simulink model "quad_eom"  (R2021a)
settings: Solver=VariableStepAuto  StartTime=0.0  StopTime=10  RelTol=1e-3
undefined symbols (not defined in the file or in its folder): eul_0, eul_init, g, I, m, pm_0, Vb_init, Vm_0, wb_init, Xe_init, xme_0
libraries: simulink_extras x3
settings Model: Creator=Petronas-Tareq  LastModifiedBy=Petronas-Tareq

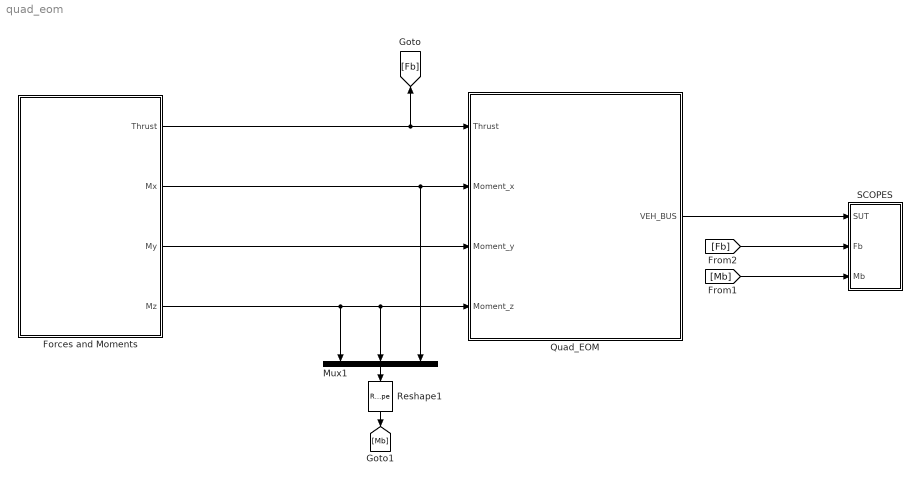
== system quad_eom ==
  Forces and Moments : Subsystem  Variant=on  VariantControlMode=label  LabelModeActiveChoice=free_fall
  Mux1 : Mux  Inputs=3
  Quad_EOM : Subsystem
      mask Display: image('$imagefile'); % Use "Edit Image" on toolstrip to change.
  Reshape1 : Reshape  OutputDimensionality=Column vector (2-D)
  SCOPES : Subsystem
  wires:
  Mux1/1 -> Reshape1/1
  Reshape1/1 -> [Mb]
  [Mb] -> SCOPES/3(Mb)
  [Fb] -> SCOPES/2(Fb)
  Quad_EOM/1(VEH_BUS) -> SCOPES/1(SUT)
  Forces and Moments/1(Thrust) -> Quad_EOM/1(Thrust), [Fb]
  Forces and Moments/2(Mx) -> Quad_EOM/2(Moment_x), Mux1/3
  Forces and Moments/3(My) -> Quad_EOM/3(Moment_y)
  Forces and Moments/4(Mz) -> Mux1/1, Quad_EOM/4(Moment_z), Mux1/2

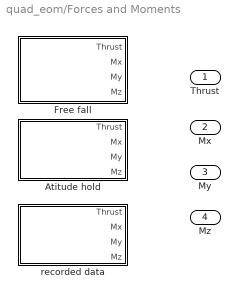
== system quad_eom/Forces and Moments ==
  Atitude hold : Subsystem  VariantControl=Alt_hold
  Free fall : Subsystem  VariantControl=free_fall
  recorded data : Subsystem  VariantControl=recorded
  Thrust : Outport
  Mx : Outport  Port=2
  My : Outport  Port=3
  Mz : Outport  Port=4

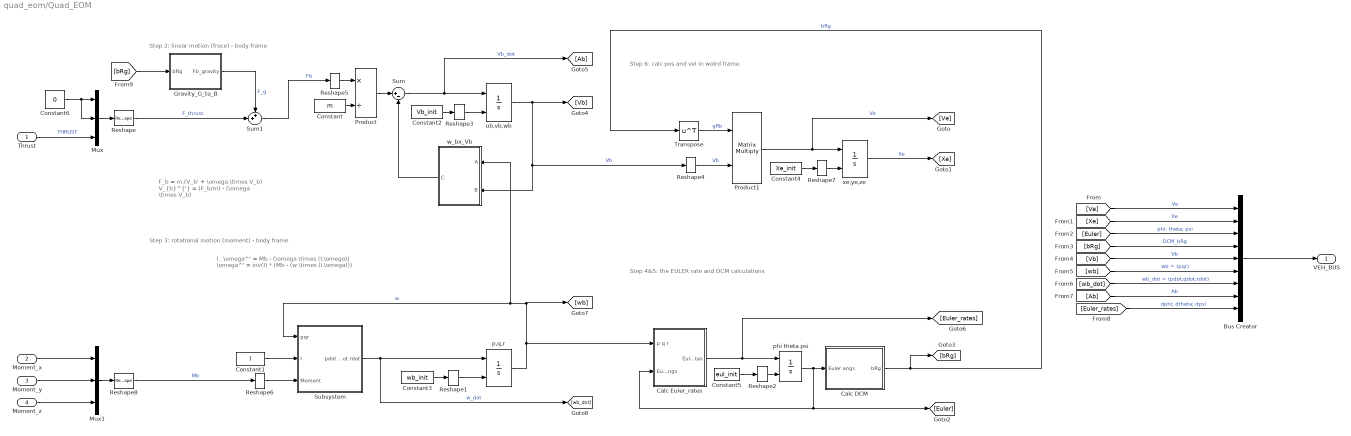
== system quad_eom/Quad_EOM ==
  note: Step 3: rotational motion (moment) - body frame
  note: F_b = m.(V_b' + \omega \times V_b)
      |
      | V_{b}^{'} = (F_b/m) - (\omega \times V_b)
  note: Step 2: linear motion (froce) - body frame
  note: Step 6: calc pos and vel in wolrd frame
  note: I . \omega^' = Mb - (\omega \times (I.\omega))
      |
      | \omega^' = inv(I) * (Mb - (w \times (I.\omega)))
  note: Step 4&5: the EULER rate and DCM calculations
  Thrust : Inport
  Moment_x : Inport  Port=2
  Moment_y : Inport  Port=3
  Moment_z : Inport  Port=4
  Bus Creator : BusCreator  Inputs=9
  Calc DCM : Subsystem
  Calc Euler_rates : Subsystem
  Constant : Constant  Value=m  OutDataTypeStr=Inherit: Inherit via back propagation
  Constant1 : Constant  Value=I  OutDataTypeStr=Inherit: Inherit via back propagation
  Constant2 : Constant  Value=Vb_init  OutDataTypeStr=Inherit: Inherit via back propagation
  Constant3 : Constant  Value=wb_init  OutDataTypeStr=Inherit: Inherit via back propagation
  Constant4 : Constant  Value=Xe_init  OutDataTypeStr=Inherit: Inherit via back propagation
  Constant5 : Constant  Value=eul_init  OutDataTypeStr=Inherit: Inherit via back propagation
  Constant6 : Constant  Value=0
  Gravity_G_to_B : Subsystem
  Mux : Mux  Inputs=3
  Mux1 : Mux  Inputs=3
  Product : Product  Inputs=*/  SaturateOnIntegerOverflow=on  OutDataTypeStr=Inherit: Same as first input
  Product1 : Product  Multiplication=Matrix(*)  InputSameDT=on  SaturateOnIntegerOverflow=on  OutDataTypeStr=Inherit: Same as first input
  Reshape{,1..8} (9 alike) : Reshape  OutputDimensionality=Column vector (2-D)
  Subsystem : Subsystem
  Sum : Sum  Inputs=|+-  SaturateOnIntegerOverflow=on
  Sum1 : Sum  Inputs=++|
  Transpose : Math  Operator=transpose  SignedPower=on  SaturateOnIntegerOverflow=on
  "p,q,r " : Integrator  InitialConditionSource=external  InitialCondition=pm_0
  phi theta psi : Integrator  InitialConditionSource=external  InitialCondition=eul_0
  ub,vb,wb : Integrator  InitialConditionSource=external  InitialCondition=Vm_0
  w_bx_Vb : Subsystem
      mask Display:
      | text(.5,.5,'Cross\nProduct\n\nC = AxB', ...
      | 	'HorizontalAlignment','Center',...
      | 	'VerticalAlignment','middle')
  xe,ye,ze : Integrator  InitialConditionSource=external  InitialCondition=xme_0
  VEH_BUS : Outport  VectorParamsAs1DForOutWhenUnconnected=off
  wires:
  [Euler] -> Bus Creator/3  "phi; theta; psi"
  [Xe] -> Bus Creator/2  "Xe"
  [Ve] -> Bus Creator/1  "Ve"
  [bRg] -> Bus Creator/4  "DCM_bRg"
  [Ab] -> Bus Creator/8  "Ab"
  [wb_dot] -> Bus Creator/7  "wb_dot = (pdot;qdot;rdot)"
  Bus Creator/1 -> VEH_BUS/1
  [Vb] -> Bus Creator/5  "Vb"
  [wb] -> Bus Creator/6  "wb = (pqr)"
  [Euler_rates] -> Bus Creator/9  "dphi; dtheta; dpsi"
  Reshape8/1 -> Reshape6/1  "Mb"
  Reshape6/1 -> Subsystem/3(Moment)
  Constant5/1 -> Reshape2/1
  Reshape1/1 -> "p,q,r "/2
  phi theta psi/1 -> Calc DCM/1(Euler angs), Calc Euler_rates/2(Euler_angs), [Euler]
  Transpose/1 -> Product1/1  "gRb"
  Constant2/1 -> Reshape3/1
  ub,vb,wb/1 -> w_bx_Vb/2(B), Reshape4/1, [Vb]  "Vb"
  Subsystem/1(pdot qdot rdot) -> [wb_dot], "p,q,r "/1  "w_dot"
  Constant/1 -> Product/2
  Constant1/1 -> Subsystem/2(I)
  Reshape4/1 -> Product1/2  "Vb"
  w_bx_Vb/1(C) -> Sum/2
  Calc DCM/1(bRg) -> [bRg], Transpose/1  "bRg"
  Calc Euler_rates/1(Euler_rates) -> [Euler_rates], phi theta psi/1
  Reshape2/1 -> phi theta psi/2
  Sum/1 -> [Ab], ub,vb,wb/1  "Vb_dot"
  Constant4/1 -> Reshape7/1
  Reshape3/1 -> ub,vb,wb/2
  "p,q,r "/1 -> [wb], Subsystem/1(pqr), w_bx_Vb/1(A), Calc Euler_rates/1("p q r ")  "w"
  Reshape7/1 -> xe,ye,ze/2
  Product1/1 -> [Ve], xe,ye,ze/1  "Ve"
  Reshape5/1 -> Product/1
  xe,ye,ze/1 -> [Xe]  "Xe"
  Sum1/1 -> Reshape5/1  "Fb"
  Constant3/1 -> Reshape1/1
  Product/1 -> Sum/1
  Constant6/1 -> Mux/2, Mux/1
  Gravity_G_to_B/1(Fb_gravity) -> Sum1/1  "F_g"
  Mux/1 -> Reshape/1
  Reshape/1 -> Sum1/2  "F_thrust"
  Thrust/1 -> Mux/3  "THRUST"
  [bRg] -> Gravity_G_to_B/1(bRg)
  Moment_y/1 -> Mux1/2
  Moment_z/1 -> Mux1/3
  Mux1/1 -> Reshape8/1
  Moment_x/1 -> Mux1/1

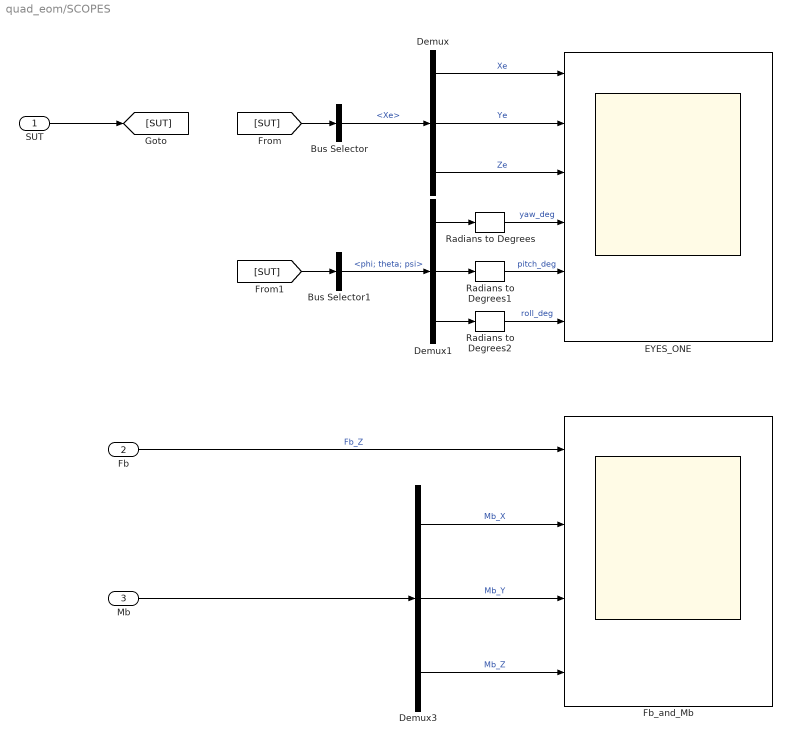
== system quad_eom/SCOPES ==
  SUT : Inport
  Fb : Inport  Port=2
  Mb : Inport  Port=3
  Bus Selector : BusSelector  OutputSignals=Xe
  Bus Selector1 : BusSelector  OutputSignals=phi; theta; psi
  Demux : Demux  Outputs=3
  Demux1 : Demux  Outputs=3
  Demux3 : Demux  Outputs=3
  EYES_ONE : Scope  NumInputPorts=6
  Fb_and_Mb : Scope  NumInputPorts=4
  Radians to Degrees : simulink_extras/Transformations/Radians to Degrees
  Radians to Degrees1 : simulink_extras/Transformations/Radians to Degrees
  Radians to Degrees2 : simulink_extras/Transformations/Radians to Degrees
  wires:
  SUT/1 -> [SUT]
  [SUT] -> Bus Selector/1
  Demux/2 -> EYES_ONE/2  "Ye"
  Demux/3 -> EYES_ONE/3  "Ze"
  Demux/1 -> EYES_ONE/1  "Xe"
  Bus Selector/1 -> Demux/1  "<Xe>"
  Bus Selector1/1 -> Demux1/1  "<phi; theta; psi>"
  [SUT] -> Bus Selector1/1
  Demux1/1 -> Radians to Degrees/1
  Radians to Degrees/1 -> EYES_ONE/4  "yaw_deg"
  Radians to Degrees1/1 -> EYES_ONE/5  "pitch_deg"
  Radians to Degrees2/1 -> EYES_ONE/6  "roll_deg"
  Demux1/3 -> Radians to Degrees2/1
  Demux1/2 -> Radians to Degrees1/1
  Fb/1 -> Fb_and_Mb/1  "Fb_Z"
  Mb/1 -> Demux3/1
  Demux3/1 -> Fb_and_Mb/2  "Mb_X"
  Demux3/2 -> Fb_and_Mb/3  "Mb_Y"
  Demux3/3 -> Fb_and_Mb/4  "Mb_Z"

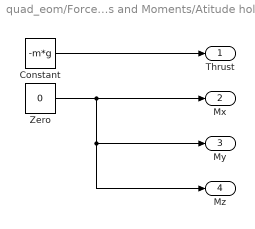
== system quad_eom/Forces and Moments/Atitude hold ==
  Constant : Constant  Value=-m*g
  Zero : Constant  Value=0  OutDataTypeStr=Inherit: Inherit via back propagation
  Thrust : Outport
  Mx : Outport  Port=2
  My : Outport  Port=3
  Mz : Outport  Port=4
  wires:
  Constant/1 -> Thrust/1
  Zero/1 -> Mz/1, My/1, Mx/1

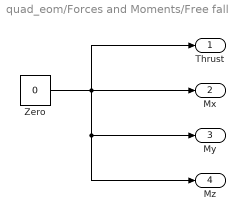
== system quad_eom/Forces and Moments/Free fall ==
  Zero : Constant  Value=0  OutDataTypeStr=Inherit: Inherit via back propagation
  Thrust : Outport
  Mx : Outport  Port=2
  My : Outport  Port=3
  Mz : Outport  Port=4
  wires:
  Zero/1 -> Thrust/1, Mx/1, My/1, Mz/1

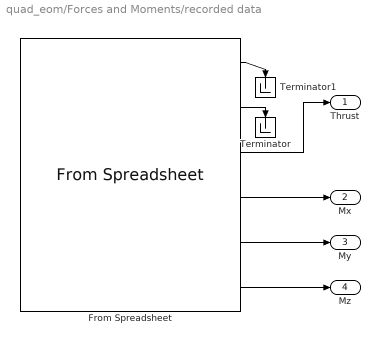
== system quad_eom/Forces and Moments/recorded data ==
  From Spreadsheet : FromSpreadsheet  FileName=FbMb_data.xlsx  SheetName=D_short_XYZ  ExtrapolationAfterLastDataPoint=Hold last value
  Terminator : Terminator
  Terminator1 : Terminator
  Thrust : Outport
  Mx : Outport  Port=2
  My : Outport  Port=3
  Mz : Outport  Port=4
  wires:
  From Spreadsheet/1 -> Terminator1/1
  From Spreadsheet/3 -> Thrust/1
  From Spreadsheet/5 -> My/1
  From Spreadsheet/2 -> Terminator/1
  From Spreadsheet/4 -> Mx/1
  From Spreadsheet/6 -> Mz/1

== system quad_eom/Quad_EOM/Calc DCM ==
  Euler angs : Inport
  Calculate DCM bRw : MATLAB Function  TreatAsAtomicUnit=on
  Demux3 : Demux  Outputs=3
  bRg : Outport
  wires:
  Calculate DCM bRw/1(bRw) -> bRg/1
  Demux3/2 -> Calculate DCM bRw/2(theta_t)  "thetsa"
  Demux3/3 -> Calculate DCM bRw/3(psi_t)  "psi"
  Demux3/1 -> Calculate DCM bRw/1(phi_t)  "phi"
  Euler angs/1 -> Demux3/1

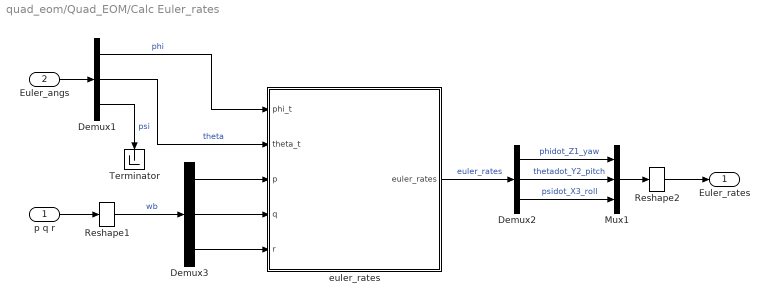
== system quad_eom/Quad_EOM/Calc Euler_rates ==
  "p q r " : Inport
  Euler_angs : Inport  Port=2
  Demux1 : Demux  Outputs=3
  Demux2 : Demux  Outputs=3
  Demux3 : Demux  Outputs=3
  Mux1 : Mux  Inputs=3
  Reshape1 : Reshape  OutputDimensionality=Column vector (2-D)
  Reshape2 : Reshape  OutputDimensionality=Column vector (2-D)
  Terminator : Terminator
  euler_rates : MATLAB Function  TreatAsAtomicUnit=on
  Euler_rates : Outport
  wires:
  Demux2/2 -> Mux1/2  "thetadot_Y2_pitch"
  Demux1/1 -> euler_rates/1(phi_t)  "phi"
  Demux3/2 -> euler_rates/4(q)
  Demux2/1 -> Mux1/1  "phidot_Z1_yaw"
  "p q r "/1 -> Reshape1/1
  Euler_angs/1 -> Demux1/1
  Demux3/1 -> euler_rates/3(p)
  Reshape2/1 -> Euler_rates/1
  Reshape1/1 -> Demux3/1  "wb"
  Demux3/3 -> euler_rates/5(r)
  Demux1/3 -> Terminator/1  "psi"
  euler_rates/1(euler_rates) -> Demux2/1  "euler_rates"
  Demux1/2 -> euler_rates/2(theta_t)  "theta"
  Mux1/1 -> Reshape2/1
  Demux2/3 -> Mux1/3  "psidot_X3_roll"

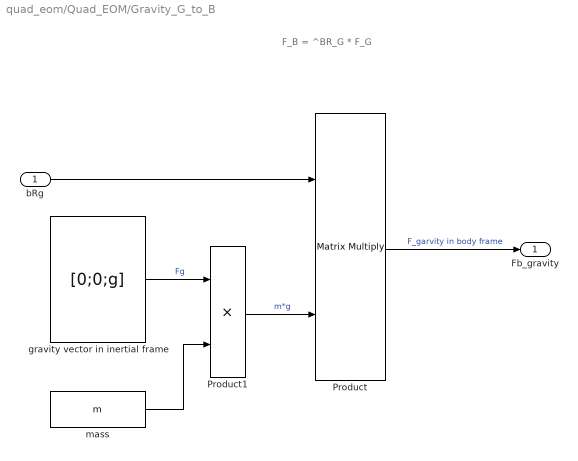
== system quad_eom/Quad_EOM/Gravity_G_to_B ==
  note: F_B = ^BR_G * F_G
  bRg : Inport
  Product : Product  Multiplication=Matrix(*)
  Product1 : Product
  gravity vector in inertial frame : Constant  Value=[0;0;g]  VectorParams1D=off
  mass : Constant  Value=m
  Fb_gravity : Outport  VectorParamsAs1DForOutWhenUnconnected=off
  wires:
  bRg/1 -> Product/1
  Product/1 -> Fb_gravity/1  "F_garvity in body frame"
  Product1/1 -> Product/2  "m*g"
  gravity vector in inertial frame/1 -> Product1/1  "Fg"
  mass/1 -> Product1/2

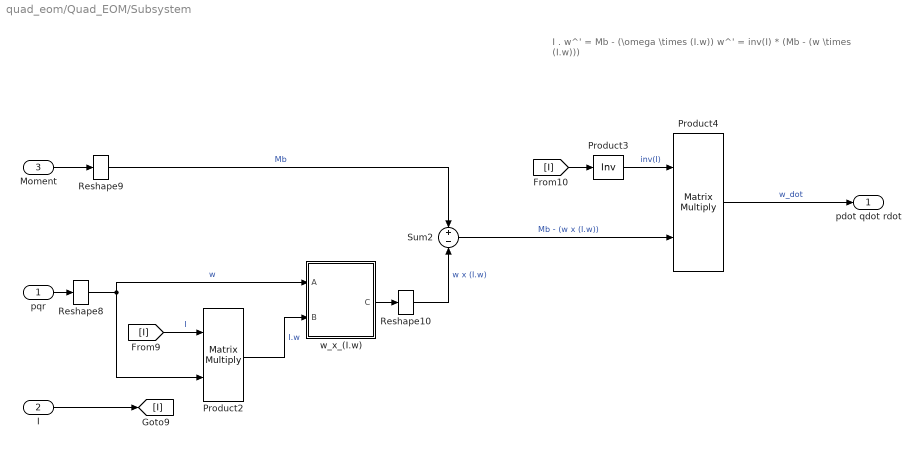
== system quad_eom/Quad_EOM/Subsystem ==
  note: I . w^' = Mb - (\omega \times (I.w))
      |
      | w^' = inv(I) * (Mb - (w \times (I.w)))
  pqr : Inport
  I : Inport  Port=2
  Moment : Inport  Port=3
  Product2 : Product  Multiplication=Matrix(*)  InputSameDT=on  SaturateOnIntegerOverflow=on  OutDataTypeStr=Inherit: Same as first input
  Product3 : Product  Inputs=/  Multiplication=Matrix(*)  SaturateOnIntegerOverflow=on  OutDataTypeStr=Inherit: Same as first input
  Product4 : Product  Multiplication=Matrix(*)  SaturateOnIntegerOverflow=on  OutDataTypeStr=Inherit: Same as first input
  Reshape10 : Reshape  OutputDimensionality=Column vector (2-D)
  Reshape8 : Reshape  OutputDimensionality=Column vector (2-D)
  Reshape9 : Reshape  OutputDimensionality=Column vector (2-D)
  Sum2 : Sum  Inputs=+|-  SaturateOnIntegerOverflow=on
  w_x_(I.w) : Subsystem
      mask Display:
      | text(.5,.5,'Cross\nProduct\n\nC = AxB', ...
      | 	'HorizontalAlignment','Center',...
      | 	'VerticalAlignment','middle')
  pdot qdot rdot : Outport
  wires:
  Product2/1 -> w_x_(I.w)/2(B)  "I.w"
  Product3/1 -> Product4/1  "inv(I)"
  Reshape8/1 -> w_x_(I.w)/1(A), Product2/2  "w"
  [I] -> Product3/1
  pqr/1 -> Reshape8/1
  Reshape9/1 -> Sum2/1  "Mb"
  Sum2/1 -> Product4/2  "Mb - (w x (I.w))"
  Reshape10/1 -> Sum2/2  "w x (I.w)"
  w_x_(I.w)/1(C) -> Reshape10/1
  [I] -> Product2/1  "I"
  Product4/1 -> pdot qdot rdot/1  "w_dot"
  Moment/1 -> Reshape9/1
  I/1 -> [I]

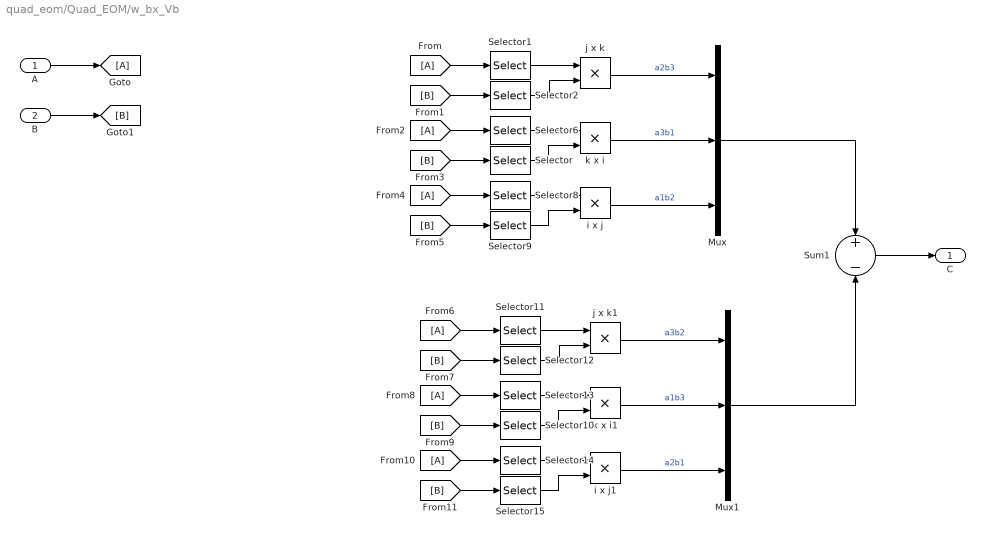
== system quad_eom/Quad_EOM/w_bx_Vb ==
  A : Inport
  B : Inport  Port=2
  Mux : Mux  Inputs=3
  Mux1 : Mux  Inputs=3
  Selector{,8,13,15} (4 alike) : Selector  InputPortWidth=3  IndexOptions=Index vector (dialog)  Indices=1  OutputSizes=1
  Selector{1,9,12,14} (4 alike) : Selector  InputPortWidth=3  IndexOptions=Index vector (dialog)  Indices=2  OutputSizes=1
  Selector{2,6,10..11} (4 alike) : Selector  InputPortWidth=3  IndexOptions=Index vector (dialog)  Indices=3  OutputSizes=1
  Sum1 : Sum  Inputs=+|-  InputSameDT=on  SaturateOnIntegerOverflow=on  OutDataTypeStr=Inherit: Same as first input
  i x j : Product  InputSameDT=on  SaturateOnIntegerOverflow=on  OutDataTypeStr=Inherit: Same as first input
  i x j1 : Product  InputSameDT=on  SaturateOnIntegerOverflow=on  OutDataTypeStr=Inherit: Same as first input
  j x k : Product  InputSameDT=on  SaturateOnIntegerOverflow=on  OutDataTypeStr=Inherit: Same as first input
  j x k1 : Product  InputSameDT=on  SaturateOnIntegerOverflow=on  OutDataTypeStr=Inherit: Same as first input
  k x i : Product  InputSameDT=on  SaturateOnIntegerOverflow=on  OutDataTypeStr=Inherit: Same as first input
  k x i1 : Product  InputSameDT=on  SaturateOnIntegerOverflow=on  OutDataTypeStr=Inherit: Same as first input
  C : Outport
  wires:
  i x j/1 -> Mux/3  "a1b2"
  k x i/1 -> Mux/2  "a3b1"
  j x k/1 -> Mux/1  "a2b3"
  Mux/1 -> Sum1/1
  Sum1/1 -> C/1
  Selector1/1 -> j x k/1
  Selector2/1 -> j x k/2
  B/1 -> [B]
  A/1 -> [A]
  [B] -> Selector2/1
  [A] -> Selector1/1
  [A] -> Selector6/1
  [B] -> Selector/1
  Selector6/1 -> k x i/1
  Selector/1 -> k x i/2
  [A] -> Selector8/1
  [B] -> Selector9/1
  Selector8/1 -> i x j/1
  Selector9/1 -> i x j/2
  i x j1/1 -> Mux1/3  "a2b1"
  k x i1/1 -> Mux1/2  "a1b3"
  j x k1/1 -> Mux1/1  "a3b2"
  Mux1/1 -> Sum1/2
  Selector11/1 -> j x k1/1
  Selector12/1 -> j x k1/2
  [B] -> Selector12/1
  [A] -> Selector11/1
  [A] -> Selector13/1
  [B] -> Selector10/1
  Selector13/1 -> k x i1/1
  Selector10/1 -> k x i1/2
  [A] -> Selector14/1
  [B] -> Selector15/1
  Selector14/1 -> i x j1/1
  Selector15/1 -> i x j1/2

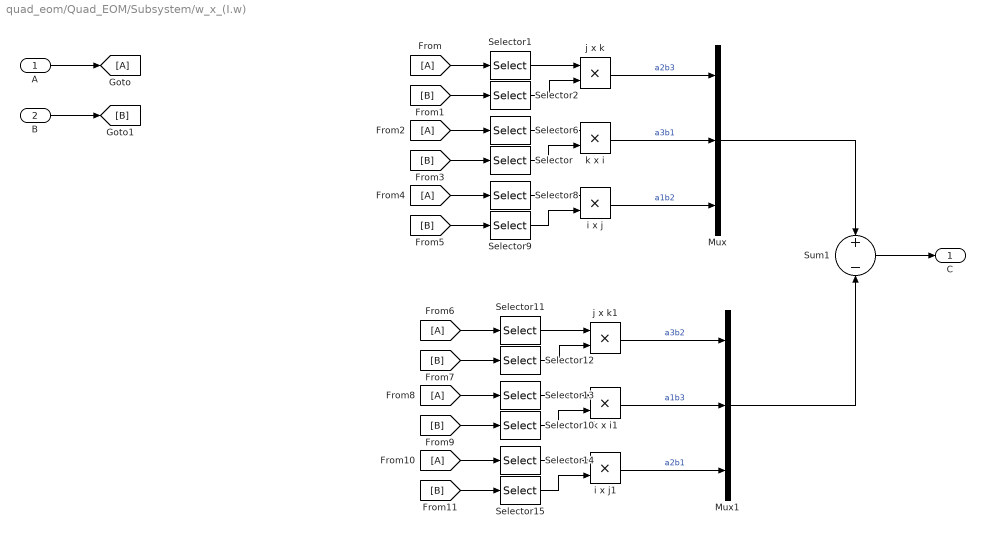
== system quad_eom/Quad_EOM/Subsystem/w_x_(I.w) ==
  A : Inport
  B : Inport  Port=2
  Mux : Mux  Inputs=3
  Mux1 : Mux  Inputs=3
  Selector{,8,13,15} (4 alike) : Selector  InputPortWidth=3  IndexOptions=Index vector (dialog)  Indices=1  OutputSizes=1
  Selector{1,9,12,14} (4 alike) : Selector  InputPortWidth=3  IndexOptions=Index vector (dialog)  Indices=2  OutputSizes=1
  Selector{2,6,10..11} (4 alike) : Selector  InputPortWidth=3  IndexOptions=Index vector (dialog)  Indices=3  OutputSizes=1
  Sum1 : Sum  Inputs=+|-  InputSameDT=on  SaturateOnIntegerOverflow=on  OutDataTypeStr=Inherit: Same as first input
  i x j : Product  InputSameDT=on  SaturateOnIntegerOverflow=on  OutDataTypeStr=Inherit: Same as first input
  i x j1 : Product  InputSameDT=on  SaturateOnIntegerOverflow=on  OutDataTypeStr=Inherit: Same as first input
  j x k : Product  InputSameDT=on  SaturateOnIntegerOverflow=on  OutDataTypeStr=Inherit: Same as first input
  j x k1 : Product  InputSameDT=on  SaturateOnIntegerOverflow=on  OutDataTypeStr=Inherit: Same as first input
  k x i : Product  InputSameDT=on  SaturateOnIntegerOverflow=on  OutDataTypeStr=Inherit: Same as first input
  k x i1 : Product  InputSameDT=on  SaturateOnIntegerOverflow=on  OutDataTypeStr=Inherit: Same as first input
  C : Outport
  wires:
  i x j/1 -> Mux/3  "a1b2"
  k x i/1 -> Mux/2  "a3b1"
  j x k/1 -> Mux/1  "a2b3"
  Mux/1 -> Sum1/1
  Sum1/1 -> C/1
  Selector1/1 -> j x k/1
  Selector2/1 -> j x k/2
  B/1 -> [B]
  A/1 -> [A]
  [B] -> Selector2/1
  [A] -> Selector1/1
  [A] -> Selector6/1
  [B] -> Selector/1
  Selector6/1 -> k x i/1
  Selector/1 -> k x i/2
  [A] -> Selector8/1
  [B] -> Selector9/1
  Selector8/1 -> i x j/1
  Selector9/1 -> i x j/2
  i x j1/1 -> Mux1/3  "a2b1"
  k x i1/1 -> Mux1/2  "a1b3"
  j x k1/1 -> Mux1/1  "a3b2"
  Mux1/1 -> Sum1/2
  Selector11/1 -> j x k1/1
  Selector12/1 -> j x k1/2
  [B] -> Selector12/1
  [A] -> Selector11/1
  [A] -> Selector13/1
  [B] -> Selector10/1
  Selector13/1 -> k x i1/1
  Selector10/1 -> k x i1/2
  [A] -> Selector14/1
  [B] -> Selector15/1
  Selector14/1 -> i x j1/1
  Selector15/1 -> i x j1/2

== matlab function quad_eom/Quad_EOM/Calc DCM/Calculate DCM bRw ==
  data: phi_t input; bRw output; theta_t input; psi_t input
function bRw = bRw(phi_t,theta_t,psi_t)
%#codegen

%    This function was generated by the Symbolic Math Toolbox version 8.7.
%    04-Nov-2022 08:55:57

bRw = reshape([cos(psi_t).*cos(theta_t),-cos(phi_t).*sin(psi_t)+cos(psi_t).*sin(phi_t).*sin(theta_t),sin(phi_t).*sin(psi_t)+cos(phi_t).*cos(psi_t).*sin(theta_t),cos(theta_t).*sin(psi_t),cos(phi_t).*cos(psi_t)+sin(phi_t).*sin(psi_t).*sin(theta_t),-cos(psi_t).*sin(phi_t)+cos(phi_t).*sin(psi_t).*sin(theta_t),-sin(theta_t),cos(theta_t).*sin(phi_t),cos(phi_t).*cos(theta_t)],[3,3]);

== matlab function quad_eom/Quad_EOM/Calc Euler_rates/euler_rates ==
  data: phi_t input; euler_rates output; theta_t input; p input; q input; r input
function euler_rates = euler_rates(phi_t,theta_t,p,q,r)
%#codegen

%    This function was generated by the Symbolic Math Toolbox version 8.7.
%    04-Nov-2022 08:55:55

euler_rates = [(p.*cos(theta_t)+r.*cos(phi_t).*sin(theta_t)+q.*sin(phi_t).*sin(theta_t))./cos(theta_t);q.*cos(phi_t)-r.*sin(phi_t);(r.*cos(phi_t)+q.*sin(phi_t))./cos(theta_t)];
